simulink model "Ass1"  (R2017a)
settings: Solver=VariableStepAuto  StartTime=0.0  StopTime=40  RelTol=1e-3
values from neighbouring files (symbols this model uses):
  B = 1    [Assingment6.m]
  J = 2    [Assingment6.m]
  J_1 = 80    [Assingment6.m]
  Kd = 39    [Assingment6.m]
  Kp = 200    [Assingment6.m]
  r = 50    [Assingment6.m]
settings Model: Creator=andersfe  LastModifiedBy=andersfe

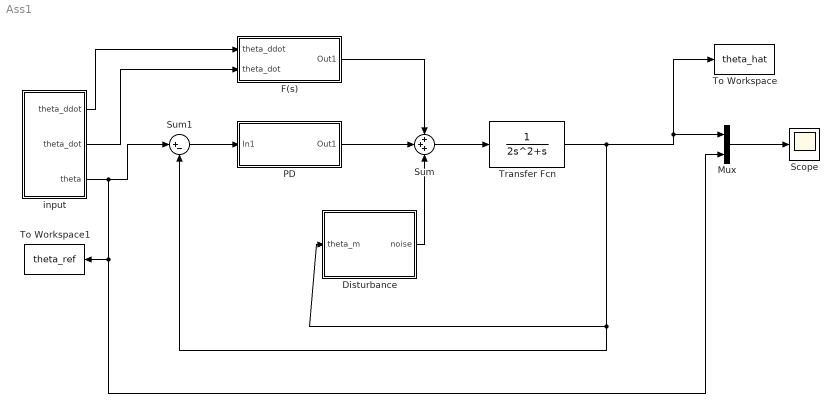
== system Ass1 ==
  Disturbance : Subsystem
  F(s) : Subsystem
  Mux : Mux  Inputs=2
  PD : Subsystem
  Scope : Scope
  Sum : Sum  Inputs=+++
  Sum1 : Sum  Inputs=|+-
  To Workspace : ToWorkspace  VariableName=theta_hat  SaveFormat=Timeseries  SampleTime=-1
  To Workspace1 : ToWorkspace  VariableName=theta_ref  SaveFormat=Timeseries  SampleTime=-1
  Transfer Fcn : TransferFcn  Denominator=[2 1 0]
  input : Subsystem
  wires:
  Sum1/1 -> PD/1(In1)
  PD/1(Out1) -> Sum/2
  F(s)/1(Out1) -> Sum/1
  Sum/1 -> Transfer Fcn/1
  Transfer Fcn/1 -> Disturbance/1("theta_m "), Sum1/2, To Workspace/1, Mux/1
  Disturbance/1("noise ") -> Sum/3
  input/3(theta) -> To Workspace1/1, Mux/2, Sum1/1
  input/1(theta_ddot) -> F(s)/1(theta_ddot)
  input/2(theta_dot) -> F(s)/2(theta_dot)
  Mux/1 -> Scope/1

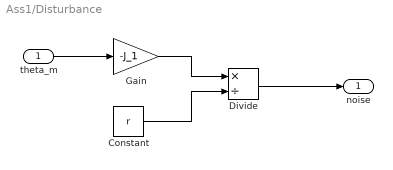
== system Ass1/Disturbance ==
  "theta_m " : Inport
  Constant : Constant  Value=r
  Divide : Product  Inputs=*/
  Gain : Gain  Gain=-J_1
  "noise " : Outport
  wires:
  "theta_m "/1 -> Gain/1
  Gain/1 -> Divide/1
  Constant/1 -> Divide/2
  Divide/1 -> "noise "/1

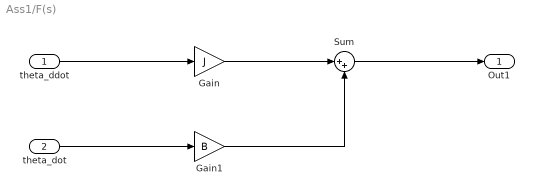
== system Ass1/F(s) ==
  theta_ddot : Inport
  theta_dot : Inport  Port=2
  Gain : Gain  Gain=J
  Gain1 : Gain  Gain=B
  Sum : Sum  Inputs=|++
  Out1 : Outport
  wires:
  theta_ddot/1 -> Gain/1
  Gain/1 -> Sum/1
  theta_dot/1 -> Gain1/1
  Gain1/1 -> Sum/2
  Sum/1 -> Out1/1

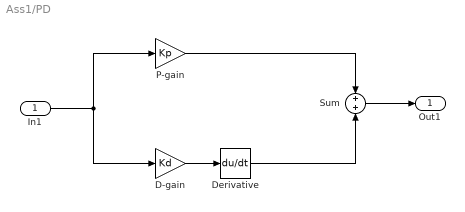
== system Ass1/PD ==
  In1 : Inport
  D-gain : Gain  Gain=Kd
  Derivative : Derivative
  P-gain : Gain  Gain=Kp
  Sum : Sum  Inputs=+|+
  Out1 : Outport
  wires:
  In1/1 -> D-gain/1, P-gain/1
  P-gain/1 -> Sum/1
  D-gain/1 -> Derivative/1
  Derivative/1 -> Sum/2
  Sum/1 -> Out1/1

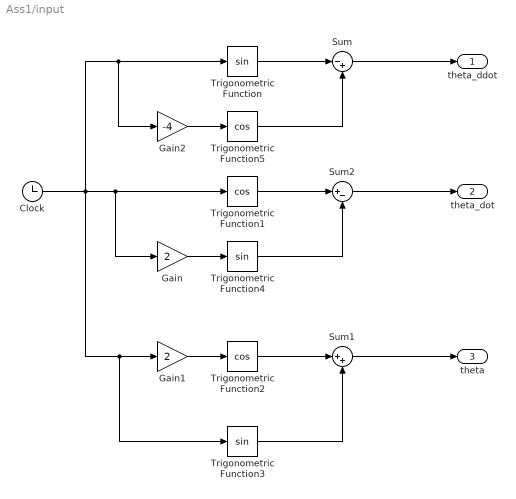
== system Ass1/input ==
  Clock : Clock
  Gain : Gain  Gain=2
  Gain1 : Gain  Gain=2
  Gain2 : Gain  Gain=-4
  Sum : Sum  Inputs=|-+
  Sum1 : Sum  Inputs=|++
  Sum2 : Sum  Inputs=|+-
  Trigonometric Function : Trigonometry
  Trigonometric Function1 : Trigonometry  Operator=cos
  Trigonometric Function2 : Trigonometry  Operator=cos
  Trigonometric Function3 : Trigonometry
  Trigonometric Function4 : Trigonometry
  Trigonometric Function5 : Trigonometry  Operator=cos
  theta_ddot : Outport
  theta_dot : Outport  Port=2
  theta : Outport  Port=3
  wires:
  Clock/1 -> Gain/1, Trigonometric Function1/1, Gain2/1, Trigonometric Function/1, Trigonometric Function3/1, Gain1/1
  Trigonometric Function/1 -> Sum/1
  Gain1/1 -> Trigonometric Function2/1
  Trigonometric Function2/1 -> Sum1/1
  Trigonometric Function3/1 -> Sum1/2
  Sum1/1 -> theta/1
  Trigonometric Function1/1 -> Sum2/1
  Gain/1 -> Trigonometric Function4/1
  Trigonometric Function4/1 -> Sum2/2
  Sum2/1 -> theta_dot/1
  Gain2/1 -> Trigonometric Function5/1
  Trigonometric Function5/1 -> Sum/2
  Sum/1 -> theta_ddot/1
